simulink model "Simulink_Observation_5"  (R2020b)
settings: Solver=VariableStepAuto  StartTime=0.0  StopTime=0  RelTol=1e-3
libraries: visionsources x1
settings Model: Creator=Mohit Akhouri  LastModifiedBy=Mohit Akhouri

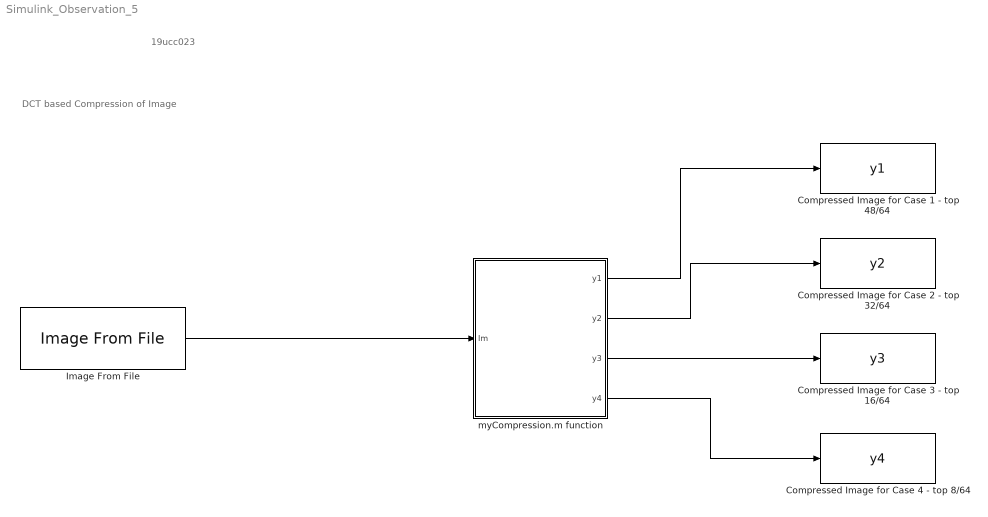
== system Simulink_Observation_5 ==
  note: DCT based Compression of Image
  note: 19ucc023
  Compressed Image for Case 1 - top 48/64 : ToWorkspace  VariableName=y1  SaveFormat=Timeseries  SampleTime=-1
  Compressed Image for Case 2 - top 32/64 : ToWorkspace  VariableName=y2  SaveFormat=Timeseries  SampleTime=-1
  Compressed Image for Case 3 - top 16/64 : ToWorkspace  VariableName=y3  SaveFormat=Timeseries  SampleTime=-1
  Compressed Image for Case 4 - top 8/64 : ToWorkspace  VariableName=y4  SaveFormat=Timeseries  SampleTime=-1
  Image From File : visionsources/Image From File  Tag=vipblks_nd  FileName=C:\Users\Mohit Akhouri\Desktop\DSP_LAB_EXP_6\cameraman.tif  Ts=inf  imagePorts=One multidimensional signal  OutPortLabels=R|G|B  ImageDataType=Inherit from input image  sdImageDataType=uint(8)  Signed=on  WordLength=16  FractionLengthMode=User-defined  FractionLength=15
  myCompression.m function : MATLAB Function  TreatAsAtomicUnit=on
  wires:
  Image From File/1 -> myCompression.m function/1(Im)
  myCompression.m function/1(y1) -> Compressed Image for Case 1 - top 48/64/1
  myCompression.m function/2(y2) -> Compressed Image for Case 2 - top 32/64/1
  myCompression.m function/3(y3) -> Compressed Image for Case 3 - top 16/64/1
  myCompression.m function/4(y4) -> Compressed Image for Case 4 - top 8/64/1

== matlab function Simulink_Observation_5/myCompression.m function ==
  data: Im input; y1 output; y2 output; y3 output; y4 output
function [y1,y2,y3,y4]  = fcn(Im)

% 19ucc023 
% Mohit Akhouri

% ALGORITHM :
% This function will compute the DCT of given image signal "Im"
% It uses the expression of "sum of cosines" to calculate the DCT

N = size(Im,1); % Size of the image (256x256)

ImF = zeros(N,N); % to store the final computed DCT

Beta = zeros(1,N); % variable that takes value 1/root(2) if i=1 else takes value 1

% algorithm for calculation of different values of variable "beta" is given
% belo , here a loop is run and correspondingly the value is set.
for i=1:N
    if i==1
        Beta(i)=1/sqrt(2);
    else
        Beta(i)=1.0;
    end
end
y1=Im;
y2=Im;
y3=Im;
y4=Im;
% Main ALGORITHM for the calculation of DCT is as follows :
for k=1:N
    for l=1:N
        sum = 0.0;
        for i=1:N
            for j=1:N
                sum = sum + (double(Im(i,j))*cos((pi*((2.0*(j-1)+1))*(k-1))/(2.0*N))*cos((pi*((2.0*(i-1))+1)*(l-1))/(2.0*N)));
            end
        end
        sum = sum * (1.0/sqrt(2.0*N)) * Beta(k) * Beta(l) ;
    end
end
